simulink model "my_robot_sim2"  (R2020a)
settings: Solver=VariableStepAuto  StartTime=0.0  StopTime=10.0  RelTol=1e-3
libraries: roblocks x4
settings Model: Creator=rusta  LastModifiedBy=rusta

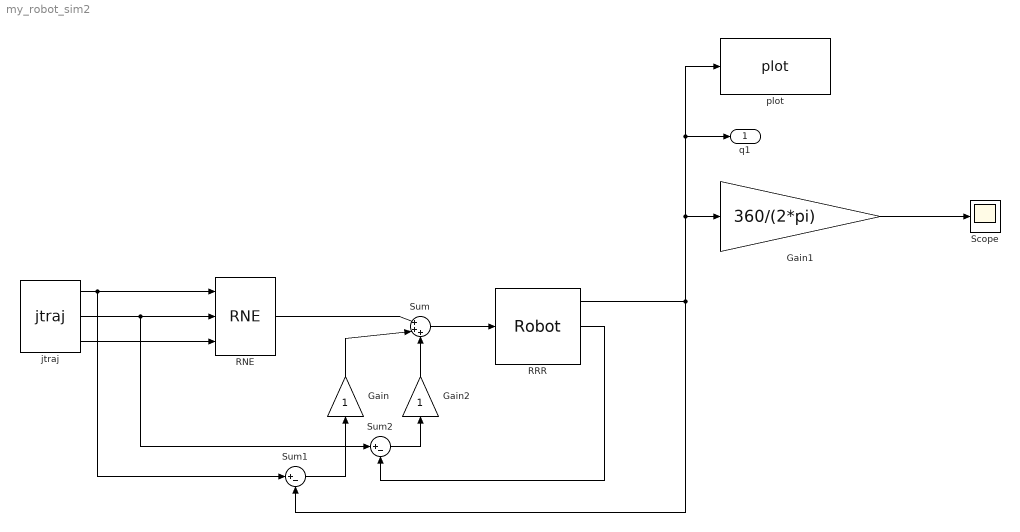
== system my_robot_sim2 ==
  Gain : Gain
  Gain1 : Gain  Gain=360/(2*pi)
  Gain2 : Gain
  RNE : roblocks/Arm/RNE  robot=rrr  grav=[0 0 9.81]
  RRR : roblocks/Arm/Robot  robot=rrr  q0=[0 0 0]
  Scope : Scope
  Sum : Sum  Inputs=|+++
  Sum1 : Sum  Inputs=|+-
  Sum2 : Sum  Inputs=|+-
  jtraj : roblocks/Toolbox/jtraj  q0=[0 0 0]  qf=[pi/2 -pi/4 -pi/4]  tmax=2  ts=0.02
  plot : roblocks/Arm/plot  robot=rrr  fps=5  holdplot=on
  q1 : Outport  VectorParamsAs1DForOutWhenUnconnected=off
  wires:
  jtraj/1 -> Sum1/1, RNE/1
  Sum2/1 -> Gain2/1
  RNE/1 -> Sum/1
  jtraj/2 -> Sum2/1, RNE/2
  jtraj/3 -> RNE/3
  RRR/2 -> Sum2/2
  Gain2/1 -> Sum/3
  RRR/1 -> plot/1, q1/1, Gain1/1, Sum1/2
  Sum1/1 -> Gain/1
  Sum/1 -> RRR/1
  Gain1/1 -> Scope/1
  Gain/1 -> Sum/2
